simulink model "PWM_v1"  (Simulink 8.5)
settings: Solver=ode23tb  StartTime=0.0  StopTime=1  MaxStep=1e-5  RelTol=1e-9
libraries: simulink x1
settings Model: Creator=Shailesh  LastModifiedBy=tesla
settings SolverCC: MaxConsecutiveMinStep=20
settings OptimizationCC: InitFltsAndDblsToZero=on
settings DebuggingCC: SaveWithParameterizedLinksMsg=none  SignalResolutionControl=TryResolveAllWithWarning  SolverPrmCheckMsg=warning  MultiTaskDSMMsg=warning  MultiTaskCondExecSysMsg=none  FcnCallInpInsideContextMsg=UseLocalSettings
settings GRTTargetCC: TargetFcnLib=ansi_tfl_tmw.mat
settings ConfigurationSet: Description=SimMechanics 2G

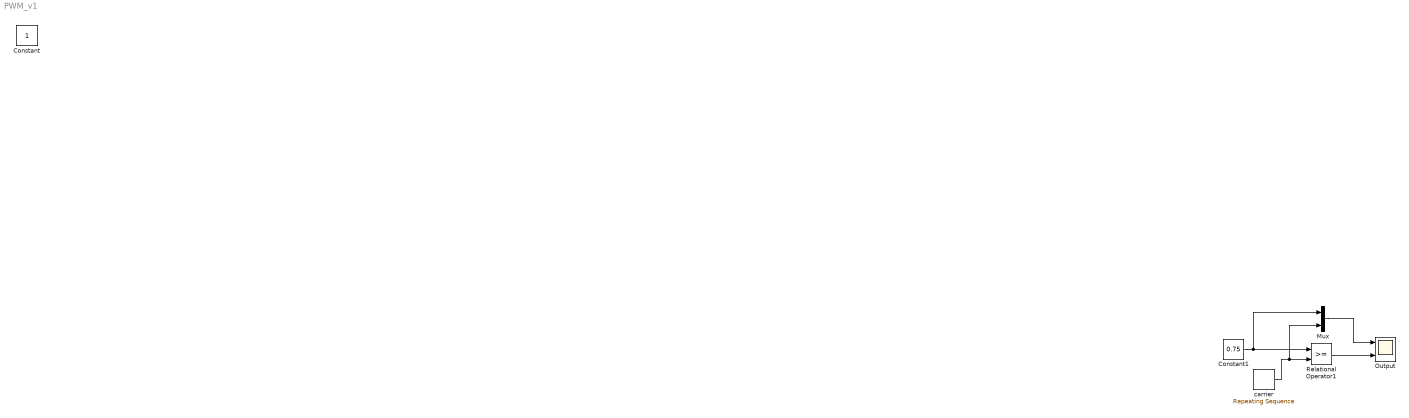
== system PWM_v1 ==
  Constant1 : Constant  Value=0.75
  Mux : Mux  Inputs=2
  Output : Scope  NumInputPorts=2
      settings: TimeRange=0.0165264352937432  YMin=-0.1~-0.1  YMax=1.1~1.1  MaxDataPoints=5000000
  Relational Operator1 : RelationalOperator  OutDataTypeStr=boolean  ZeroCross=off
  carrier : simulink/Sources/Repeating Sequence  rep_seq_t=[0 1/1e3]  rep_seq_y=[0 1]
  Constant : Constant  IOType=siggen
  wires:
  Relational Operator1/1 -> Output/2
  carrier/1 -> Mux/2, Relational Operator1/2
  Constant1/1 -> Mux/1, Relational Operator1/1
  Mux/1 -> Output/1
